simulink model "six_plus_six_AcmsteeringV09_main_1lf"  (R2014a)
settings: Solver=FixedStepDiscrete  StartTime=0.0  StopTime=10.0  FixedStep=0.0005  RelTol=1e-3
InitFcn:
  | Veh_Par_wxt
undefined symbols (not defined in the file or in its folder): acc_spdctl, ag_thr, B, bra_em, bra_pre_gz2, bra_pre_gz34, bra_pre_yd, brakepre_dem_data, brakeTrq_dem_data, bratrq_max, ecucoder_acal, eff_tran, ESP_switch, G, guzhang_lf, guzhang_lm, guzhang_lr, guzhang_rf, guzhang_rm, guzhang_rr, kd1, kd2, ki1, ki2, kp1, kp2, L, myFIS, premax, Radius, RC_switch, s_opt_yi, s_opt_zhuan, s_opt_zhuan_add, s_opt_zhuan_table, spd_map_mot, spd_spdctl, speed_thr_park, TCS_switch, tras_ratio, trq_map_mot, trqmax_yd, trqmax_zx, trqmaxneg, v_gain, v_table, v_thr_park, zhidong_bianmazhi, zhidong_down, zhidong_up, zhidong_youmen, zhuanxiang_bianmazhi, zhuanxiang_down, zhuanxiang_up, zhuanxiang_youmen
libraries: simulink x980, ec5744lib x59, fuzblock x2
(part 5 of 25)

== system six_plus_six_AcmsteeringV09_main_1lf/Data_input/BMS1-2/BMS1 ==
  input : Inport
  Enable : EnablePort
  BMS1_SOC_Ad : Sum
  BMS1_SOC_Convert : DataTypeConversion  OutDataTypeStr=uint32
  BMS1_SOC_F : Gain  Gain=0.1
  BMS1_SOC_L : simulink/Logic and Bit Operations/Bitwise Operator  logicop=AND  UseBitMask=on  BitMask=65535  BitMaskRealWorld=Stored Integer
  BMS1_SOC_O : Constant  Value=0  OutDataTypeStr=single
  BMS1_SOC_S : ArithShift
  BMS1_SOC_Sub : Subsystem
  BMS1_SOC_sat : Saturate  UpperLimit=1000  LowerLimit=0
  BMS1_SOCcv : DataTypeConversion
  BMS1_SOCinput5_Ad : Sum
  BMS1_SOCinput5_C : Constant  Value=256
  BMS1_SOCinput5_P : Product
  BMS1_Sys_Status1_Ad : Sum
  BMS1_Sys_Status1_Convert : DataTypeConversion  OutDataTypeStr=uint32
  BMS1_Sys_Status1_F : Gain
  BMS1_Sys_Status1_L : simulink/Logic and Bit Operations/Bitwise Operator  logicop=AND  UseBitMask=on  BitMask=255  BitMaskRealWorld=Stored Integer
  BMS1_Sys_Status1_O : Constant  Value=0  OutDataTypeStr=single
  BMS1_Sys_Status1_S : ArithShift
  BMS1_Sys_Status1_Sub : Subsystem
  BMS1_Sys_Status1_sat : Saturate  UpperLimit=255  LowerLimit=0
  BMS1_Sys_Status1cv : DataTypeConversion
  BMS1_Sys_Status2_Ad : Sum
  BMS1_Sys_Status2_Convert : DataTypeConversion  OutDataTypeStr=uint32
  BMS1_Sys_Status2_F : Gain
  BMS1_Sys_Status2_L : simulink/Logic and Bit Operations/Bitwise Operator  logicop=AND  UseBitMask=on  BitMask=255  BitMaskRealWorld=Stored Integer
  BMS1_Sys_Status2_O : Constant  Value=0  OutDataTypeStr=single
  BMS1_Sys_Status2_S : ArithShift
  BMS1_Sys_Status2_Sub : Subsystem
  BMS1_Sys_Status2_sat : Saturate  UpperLimit=255  LowerLimit=0
  BMS1_Sys_Status2cv : DataTypeConversion
  BMS1_TotalCurrent_Ad : Sum
  BMS1_TotalCurrent_Convert : DataTypeConversion  OutDataTypeStr=uint32
  BMS1_TotalCurrent_F : Gain  Gain=0.1
  BMS1_TotalCurrent_L : simulink/Logic and Bit Operations/Bitwise Operator  logicop=AND  UseBitMask=on  BitMask=65535  BitMaskRealWorld=Stored Integer
  BMS1_TotalCurrent_O : Constant  Value=-32000  OutDataTypeStr=single
  BMS1_TotalCurrent_S : ArithShift
  BMS1_TotalCurrent_Sub : Subsystem
  BMS1_TotalCurrent_sat : Saturate  UpperLimit=3353.5  LowerLimit=-32000
  BMS1_TotalCurrentcv : DataTypeConversion
  BMS1_TotalCurrentinput3_Ad : Sum
  BMS1_TotalCurrentinput3_C : Constant  Value=256
  BMS1_TotalCurrentinput3_P : Product
  BMS1_TotalVol_Ad : Sum
  BMS1_TotalVol_Convert : DataTypeConversion  OutDataTypeStr=uint32
  BMS1_TotalVol_F : Gain  Gain=0.1
  BMS1_TotalVol_L : simulink/Logic and Bit Operations/Bitwise Operator  logicop=AND  UseBitMask=on  BitMask=65535  BitMaskRealWorld=Stored Integer
  BMS1_TotalVol_O : Constant  Value=0  OutDataTypeStr=single
  BMS1_TotalVol_S : ArithShift
  BMS1_TotalVol_Sub : Subsystem
  BMS1_TotalVol_sat : Saturate  UpperLimit=6553.5  LowerLimit=0
  BMS1_TotalVolcv : DataTypeConversion
  BMS1_TotalVolinput1_Ad : Sum
  BMS1_TotalVolinput1_C : Constant  Value=256
  BMS1_TotalVolinput1_P : Product
  Demux : Demux  Outputs=8
  BMS1_TotalVol_Out : Outport
  BMS1_TotalCurrent_Out : Outport  Port=2
  BMS1_Sys_Status2_Out : Outport  Port=3
  BMS1_Sys_Status1_Out : Outport  Port=4
  BMS1_SOC_Out : Outport  Port=5
  wires:
  BMS1_TotalVol_F/1 -> BMS1_TotalVol_Ad/1
  BMS1_TotalVol_O/1 -> BMS1_TotalVol_Ad/2
  BMS1_TotalVol_Ad/1 -> BMS1_TotalVol_sat/1
  BMS1_TotalVol_sat/1 -> BMS1_TotalVol_Out/1
  Demux/1 -> BMS1_TotalVolinput1_P/1
  BMS1_TotalVolinput1_C/1 -> BMS1_TotalVolinput1_P/2
  BMS1_TotalVolinput1_P/1 -> BMS1_TotalVolinput1_Ad/1
  Demux/2 -> BMS1_TotalVolinput1_Ad/2
  BMS1_TotalVolinput1_Ad/1 -> BMS1_TotalVol_Sub/1(In1)
  BMS1_TotalVol_Sub/1(Out1) -> BMS1_TotalVol_Convert/1
  BMS1_TotalVol_Convert/1 -> BMS1_TotalVol_L/1
  BMS1_TotalVol_L/1 -> BMS1_TotalVol_S/1
  BMS1_TotalVol_S/1 -> BMS1_TotalVolcv/1
  BMS1_TotalVolcv/1 -> BMS1_TotalVol_F/1
  BMS1_TotalCurrent_F/1 -> BMS1_TotalCurrent_Ad/1
  BMS1_TotalCurrent_O/1 -> BMS1_TotalCurrent_Ad/2
  BMS1_TotalCurrent_Ad/1 -> BMS1_TotalCurrent_sat/1
  BMS1_TotalCurrent_sat/1 -> BMS1_TotalCurrent_Out/1
  Demux/3 -> BMS1_TotalCurrentinput3_P/1
  BMS1_TotalCurrentinput3_C/1 -> BMS1_TotalCurrentinput3_P/2
  BMS1_TotalCurrentinput3_P/1 -> BMS1_TotalCurrentinput3_Ad/1
  Demux/4 -> BMS1_TotalCurrentinput3_Ad/2
  BMS1_TotalCurrentinput3_Ad/1 -> BMS1_TotalCurrent_Sub/1(In1)
  BMS1_TotalCurrent_Sub/1(Out1) -> BMS1_TotalCurrent_Convert/1
  BMS1_TotalCurrent_Convert/1 -> BMS1_TotalCurrent_L/1
  BMS1_TotalCurrent_L/1 -> BMS1_TotalCurrent_S/1
  BMS1_TotalCurrent_S/1 -> BMS1_TotalCurrentcv/1
  BMS1_TotalCurrentcv/1 -> BMS1_TotalCurrent_F/1
  BMS1_Sys_Status2_F/1 -> BMS1_Sys_Status2_Ad/1
  BMS1_Sys_Status2_O/1 -> BMS1_Sys_Status2_Ad/2
  BMS1_Sys_Status2_Ad/1 -> BMS1_Sys_Status2_sat/1
  BMS1_Sys_Status2_sat/1 -> BMS1_Sys_Status2_Out/1
  Demux/8 -> BMS1_Sys_Status2_Sub/1(In1)
  BMS1_Sys_Status2_Sub/1(Out1) -> BMS1_Sys_Status2_Convert/1
  BMS1_Sys_Status2_Convert/1 -> BMS1_Sys_Status2_L/1
  BMS1_Sys_Status2_L/1 -> BMS1_Sys_Status2_S/1
  BMS1_Sys_Status2_S/1 -> BMS1_Sys_Status2cv/1
  BMS1_Sys_Status2cv/1 -> BMS1_Sys_Status2_F/1
  BMS1_Sys_Status1_F/1 -> BMS1_Sys_Status1_Ad/1
  BMS1_Sys_Status1_O/1 -> BMS1_Sys_Status1_Ad/2
  BMS1_Sys_Status1_Ad/1 -> BMS1_Sys_Status1_sat/1
  BMS1_Sys_Status1_sat/1 -> BMS1_Sys_Status1_Out/1
  Demux/7 -> BMS1_Sys_Status1_Sub/1(In1)
  BMS1_Sys_Status1_Sub/1(Out1) -> BMS1_Sys_Status1_Convert/1
  BMS1_Sys_Status1_Convert/1 -> BMS1_Sys_Status1_L/1
  BMS1_Sys_Status1_L/1 -> BMS1_Sys_Status1_S/1
  BMS1_Sys_Status1_S/1 -> BMS1_Sys_Status1cv/1
  BMS1_Sys_Status1cv/1 -> BMS1_Sys_Status1_F/1
  BMS1_SOC_F/1 -> BMS1_SOC_Ad/1
  BMS1_SOC_O/1 -> BMS1_SOC_Ad/2
  BMS1_SOC_Ad/1 -> BMS1_SOC_sat/1
  BMS1_SOC_sat/1 -> BMS1_SOC_Out/1
  Demux/5 -> BMS1_SOCinput5_P/1
  BMS1_SOCinput5_C/1 -> BMS1_SOCinput5_P/2
  BMS1_SOCinput5_P/1 -> BMS1_SOCinput5_Ad/1
  Demux/6 -> BMS1_SOCinput5_Ad/2
  BMS1_SOCinput5_Ad/1 -> BMS1_SOC_Sub/1(In1)
  BMS1_SOC_Sub/1(Out1) -> BMS1_SOC_Convert/1
  BMS1_SOC_Convert/1 -> BMS1_SOC_L/1
  BMS1_SOC_L/1 -> BMS1_SOC_S/1
  BMS1_SOC_S/1 -> BMS1_SOCcv/1
  BMS1_SOCcv/1 -> BMS1_SOC_F/1
  input/1 -> Demux/1

== system six_plus_six_AcmsteeringV09_main_1lf/Data_input/BMS1_1/BMS1 ==
  input : Inport
  Enable : EnablePort
  BMS1_SOC_Ad : Sum
  BMS1_SOC_Convert : DataTypeConversion  OutDataTypeStr=uint32
  BMS1_SOC_F : Gain  Gain=0.1
  BMS1_SOC_L : simulink/Logic and Bit Operations/Bitwise Operator  logicop=AND  UseBitMask=on  BitMask=65535  BitMaskRealWorld=Stored Integer
  BMS1_SOC_O : Constant  Value=0  OutDataTypeStr=single
  BMS1_SOC_S : ArithShift
  BMS1_SOC_Sub : Subsystem
  BMS1_SOC_sat : Saturate  UpperLimit=1000  LowerLimit=0
  BMS1_SOCcv : DataTypeConversion
  BMS1_SOCinput5_Ad : Sum
  BMS1_SOCinput5_C : Constant  Value=256
  BMS1_SOCinput5_P : Product
  BMS1_Sys_Status1_Ad : Sum
  BMS1_Sys_Status1_Convert : DataTypeConversion  OutDataTypeStr=uint32
  BMS1_Sys_Status1_F : Gain
  BMS1_Sys_Status1_L : simulink/Logic and Bit Operations/Bitwise Operator  logicop=AND  UseBitMask=on  BitMask=255  BitMaskRealWorld=Stored Integer
  BMS1_Sys_Status1_O : Constant  Value=0  OutDataTypeStr=single
  BMS1_Sys_Status1_S : ArithShift
  BMS1_Sys_Status1_Sub : Subsystem
  BMS1_Sys_Status1_sat : Saturate  UpperLimit=255  LowerLimit=0
  BMS1_Sys_Status1cv : DataTypeConversion
  BMS1_Sys_Status2_Ad : Sum
  BMS1_Sys_Status2_Convert : DataTypeConversion  OutDataTypeStr=uint32
  BMS1_Sys_Status2_F : Gain
  BMS1_Sys_Status2_L : simulink/Logic and Bit Operations/Bitwise Operator  logicop=AND  UseBitMask=on  BitMask=255  BitMaskRealWorld=Stored Integer
  BMS1_Sys_Status2_O : Constant  Value=0  OutDataTypeStr=single
  BMS1_Sys_Status2_S : ArithShift
  BMS1_Sys_Status2_Sub : Subsystem
  BMS1_Sys_Status2_sat : Saturate  UpperLimit=255  LowerLimit=0
  BMS1_Sys_Status2cv : DataTypeConversion
  BMS1_TotalCurrent_Ad : Sum
  BMS1_TotalCurrent_Convert : DataTypeConversion  OutDataTypeStr=uint32
  BMS1_TotalCurrent_F : Gain  Gain=0.1
  BMS1_TotalCurrent_L : simulink/Logic and Bit Operations/Bitwise Operator  logicop=AND  UseBitMask=on  BitMask=65535  BitMaskRealWorld=Stored Integer
  BMS1_TotalCurrent_O : Constant  Value=-32000  OutDataTypeStr=single
  BMS1_TotalCurrent_S : ArithShift
  BMS1_TotalCurrent_Sub : Subsystem
  BMS1_TotalCurrent_sat : Saturate  UpperLimit=3353.5  LowerLimit=-32000
  BMS1_TotalCurrentcv : DataTypeConversion
  BMS1_TotalCurrentinput3_Ad : Sum
  BMS1_TotalCurrentinput3_C : Constant  Value=256
  BMS1_TotalCurrentinput3_P : Product
  BMS1_TotalVol_Ad : Sum
  BMS1_TotalVol_Convert : DataTypeConversion  OutDataTypeStr=uint32
  BMS1_TotalVol_F : Gain  Gain=0.1
  BMS1_TotalVol_L : simulink/Logic and Bit Operations/Bitwise Operator  logicop=AND  UseBitMask=on  BitMask=65535  BitMaskRealWorld=Stored Integer
  BMS1_TotalVol_O : Constant  Value=0  OutDataTypeStr=single
  BMS1_TotalVol_S : ArithShift
  BMS1_TotalVol_Sub : Subsystem
  BMS1_TotalVol_sat : Saturate  UpperLimit=6553.5  LowerLimit=0
  BMS1_TotalVolcv : DataTypeConversion
  BMS1_TotalVolinput1_Ad : Sum
  BMS1_TotalVolinput1_C : Constant  Value=256
  BMS1_TotalVolinput1_P : Product
  Demux : Demux  Outputs=8
  BMS1_TotalVol_Out : Outport
  BMS1_TotalCurrent_Out : Outport  Port=2
  BMS1_Sys_Status2_Out : Outport  Port=3
  BMS1_Sys_Status1_Out : Outport  Port=4
  BMS1_SOC_Out : Outport  Port=5
  wires:
  BMS1_TotalVol_F/1 -> BMS1_TotalVol_Ad/1
  BMS1_TotalVol_O/1 -> BMS1_TotalVol_Ad/2
  BMS1_TotalVol_Ad/1 -> BMS1_TotalVol_sat/1
  BMS1_TotalVol_sat/1 -> BMS1_TotalVol_Out/1
  Demux/1 -> BMS1_TotalVolinput1_P/1
  BMS1_TotalVolinput1_C/1 -> BMS1_TotalVolinput1_P/2
  BMS1_TotalVolinput1_P/1 -> BMS1_TotalVolinput1_Ad/1
  Demux/2 -> BMS1_TotalVolinput1_Ad/2
  BMS1_TotalVolinput1_Ad/1 -> BMS1_TotalVol_Sub/1(In1)
  BMS1_TotalVol_Sub/1(Out1) -> BMS1_TotalVol_Convert/1
  BMS1_TotalVol_Convert/1 -> BMS1_TotalVol_L/1
  BMS1_TotalVol_L/1 -> BMS1_TotalVol_S/1
  BMS1_TotalVol_S/1 -> BMS1_TotalVolcv/1
  BMS1_TotalVolcv/1 -> BMS1_TotalVol_F/1
  BMS1_TotalCurrent_F/1 -> BMS1_TotalCurrent_Ad/1
  BMS1_TotalCurrent_O/1 -> BMS1_TotalCurrent_Ad/2
  BMS1_TotalCurrent_Ad/1 -> BMS1_TotalCurrent_sat/1
  BMS1_TotalCurrent_sat/1 -> BMS1_TotalCurrent_Out/1
  Demux/3 -> BMS1_TotalCurrentinput3_P/1
  BMS1_TotalCurrentinput3_C/1 -> BMS1_TotalCurrentinput3_P/2
  BMS1_TotalCurrentinput3_P/1 -> BMS1_TotalCurrentinput3_Ad/1
  Demux/4 -> BMS1_TotalCurrentinput3_Ad/2
  BMS1_TotalCurrentinput3_Ad/1 -> BMS1_TotalCurrent_Sub/1(In1)
  BMS1_TotalCurrent_Sub/1(Out1) -> BMS1_TotalCurrent_Convert/1
  BMS1_TotalCurrent_Convert/1 -> BMS1_TotalCurrent_L/1
  BMS1_TotalCurrent_L/1 -> BMS1_TotalCurrent_S/1
  BMS1_TotalCurrent_S/1 -> BMS1_TotalCurrentcv/1
  BMS1_TotalCurrentcv/1 -> BMS1_TotalCurrent_F/1
  BMS1_Sys_Status2_F/1 -> BMS1_Sys_Status2_Ad/1
  BMS1_Sys_Status2_O/1 -> BMS1_Sys_Status2_Ad/2
  BMS1_Sys_Status2_Ad/1 -> BMS1_Sys_Status2_sat/1
  BMS1_Sys_Status2_sat/1 -> BMS1_Sys_Status2_Out/1
  Demux/8 -> BMS1_Sys_Status2_Sub/1(In1)
  BMS1_Sys_Status2_Sub/1(Out1) -> BMS1_Sys_Status2_Convert/1
  BMS1_Sys_Status2_Convert/1 -> BMS1_Sys_Status2_L/1
  BMS1_Sys_Status2_L/1 -> BMS1_Sys_Status2_S/1
  BMS1_Sys_Status2_S/1 -> BMS1_Sys_Status2cv/1
  BMS1_Sys_Status2cv/1 -> BMS1_Sys_Status2_F/1
  BMS1_Sys_Status1_F/1 -> BMS1_Sys_Status1_Ad/1
  BMS1_Sys_Status1_O/1 -> BMS1_Sys_Status1_Ad/2
  BMS1_Sys_Status1_Ad/1 -> BMS1_Sys_Status1_sat/1
  BMS1_Sys_Status1_sat/1 -> BMS1_Sys_Status1_Out/1
  Demux/7 -> BMS1_Sys_Status1_Sub/1(In1)
  BMS1_Sys_Status1_Sub/1(Out1) -> BMS1_Sys_Status1_Convert/1
  BMS1_Sys_Status1_Convert/1 -> BMS1_Sys_Status1_L/1
  BMS1_Sys_Status1_L/1 -> BMS1_Sys_Status1_S/1
  BMS1_Sys_Status1_S/1 -> BMS1_Sys_Status1cv/1
  BMS1_Sys_Status1cv/1 -> BMS1_Sys_Status1_F/1
  BMS1_SOC_F/1 -> BMS1_SOC_Ad/1
  BMS1_SOC_O/1 -> BMS1_SOC_Ad/2
  BMS1_SOC_Ad/1 -> BMS1_SOC_sat/1
  BMS1_SOC_sat/1 -> BMS1_SOC_Out/1
  Demux/5 -> BMS1_SOCinput5_P/1
  BMS1_SOCinput5_C/1 -> BMS1_SOCinput5_P/2
  BMS1_SOCinput5_P/1 -> BMS1_SOCinput5_Ad/1
  Demux/6 -> BMS1_SOCinput5_Ad/2
  BMS1_SOCinput5_Ad/1 -> BMS1_SOC_Sub/1(In1)
  BMS1_SOC_Sub/1(Out1) -> BMS1_SOC_Convert/1
  BMS1_SOC_Convert/1 -> BMS1_SOC_L/1
  BMS1_SOC_L/1 -> BMS1_SOC_S/1
  BMS1_SOC_S/1 -> BMS1_SOCcv/1
  BMS1_SOCcv/1 -> BMS1_SOC_F/1
  input/1 -> Demux/1

== system six_plus_six_AcmsteeringV09_main_1lf/Data_input/BMS2/BMS2 ==
  input : Inport
  Enable : EnablePort
  BMS2_HighSingleVol_Ad : Sum
  BMS2_HighSingleVol_Convert : DataTypeConversion  OutDataTypeStr=uint32
  BMS2_HighSingleVol_F : Gain
  BMS2_HighSingleVol_L : simulink/Logic and Bit Operations/Bitwise Operator  logicop=AND  UseBitMask=on  BitMask=65535  BitMaskRealWorld=Stored Integer
  BMS2_HighSingleVol_O : Constant  Value=0  OutDataTypeStr=single
  BMS2_HighSingleVol_S : ArithShift
  BMS2_HighSingleVol_Sub : Subsystem
  BMS2_HighSingleVol_sat : Saturate  UpperLimit=10  LowerLimit=0
  BMS2_HighSingleVolcv : DataTypeConversion
  BMS2_HighSingleVolinput1_Ad : Sum
  BMS2_HighSingleVolinput1_C : Constant  Value=256
  BMS2_HighSingleVolinput1_P : Product
  BMS2_LowSingleVol_Ad : Sum
  BMS2_LowSingleVol_Convert : DataTypeConversion  OutDataTypeStr=uint32
  BMS2_LowSingleVol_F : Gain
  BMS2_LowSingleVol_L : simulink/Logic and Bit Operations/Bitwise Operator  logicop=AND  UseBitMask=on  BitMask=65535  BitMaskRealWorld=Stored Integer
  BMS2_LowSingleVol_O : Constant  Value=0  OutDataTypeStr=single
  BMS2_LowSingleVol_S : ArithShift
  BMS2_LowSingleVol_Sub : Subsystem
  BMS2_LowSingleVol_sat : Saturate  UpperLimit=65535  LowerLimit=0
  BMS2_LowSingleVolcv : DataTypeConversion
  BMS2_LowSingleVolinput3_Ad : Sum
  BMS2_LowSingleVolinput3_C : Constant  Value=256
  BMS2_LowSingleVolinput3_P : Product
  Demux : Demux  Outputs=8
  BMS2_LowSingleVol_Out : Outport
  BMS2_HighSingleVol_Out : Outport  Port=2
  wires:
  BMS2_LowSingleVol_F/1 -> BMS2_LowSingleVol_Ad/1
  BMS2_LowSingleVol_O/1 -> BMS2_LowSingleVol_Ad/2
  BMS2_LowSingleVol_Ad/1 -> BMS2_LowSingleVol_sat/1
  BMS2_LowSingleVol_sat/1 -> BMS2_LowSingleVol_Out/1
  Demux/3 -> BMS2_LowSingleVolinput3_P/1
  BMS2_LowSingleVolinput3_C/1 -> BMS2_LowSingleVolinput3_P/2
  BMS2_LowSingleVolinput3_P/1 -> BMS2_LowSingleVolinput3_Ad/1
  Demux/4 -> BMS2_LowSingleVolinput3_Ad/2
  BMS2_LowSingleVolinput3_Ad/1 -> BMS2_LowSingleVol_Sub/1(In1)
  BMS2_LowSingleVol_Sub/1(Out1) -> BMS2_LowSingleVol_Convert/1
  BMS2_LowSingleVol_Convert/1 -> BMS2_LowSingleVol_L/1
  BMS2_LowSingleVol_L/1 -> BMS2_LowSingleVol_S/1
  BMS2_LowSingleVol_S/1 -> BMS2_LowSingleVolcv/1
  BMS2_LowSingleVolcv/1 -> BMS2_LowSingleVol_F/1
  BMS2_HighSingleVol_F/1 -> BMS2_HighSingleVol_Ad/1
  BMS2_HighSingleVol_O/1 -> BMS2_HighSingleVol_Ad/2
  BMS2_HighSingleVol_Ad/1 -> BMS2_HighSingleVol_sat/1
  BMS2_HighSingleVol_sat/1 -> BMS2_HighSingleVol_Out/1
  Demux/1 -> BMS2_HighSingleVolinput1_P/1
  BMS2_HighSingleVolinput1_C/1 -> BMS2_HighSingleVolinput1_P/2
  BMS2_HighSingleVolinput1_P/1 -> BMS2_HighSingleVolinput1_Ad/1
  Demux/2 -> BMS2_HighSingleVolinput1_Ad/2
  BMS2_HighSingleVolinput1_Ad/1 -> BMS2_HighSingleVol_Sub/1(In1)
  BMS2_HighSingleVol_Sub/1(Out1) -> BMS2_HighSingleVol_Convert/1
  BMS2_HighSingleVol_Convert/1 -> BMS2_HighSingleVol_L/1
  BMS2_HighSingleVol_L/1 -> BMS2_HighSingleVol_S/1
  BMS2_HighSingleVol_S/1 -> BMS2_HighSingleVolcv/1
  BMS2_HighSingleVolcv/1 -> BMS2_HighSingleVol_F/1
  input/1 -> Demux/1

== system six_plus_six_AcmsteeringV09_main_1lf/Data_input/BMS2_1/BMS2 ==
  input : Inport
  Enable : EnablePort
  BMS2_HighSingleVol_Ad : Sum
  BMS2_HighSingleVol_Convert : DataTypeConversion  OutDataTypeStr=uint32
  BMS2_HighSingleVol_F : Gain
  BMS2_HighSingleVol_L : simulink/Logic and Bit Operations/Bitwise Operator  logicop=AND  UseBitMask=on  BitMask=65535  BitMaskRealWorld=Stored Integer
  BMS2_HighSingleVol_O : Constant  Value=0  OutDataTypeStr=single
  BMS2_HighSingleVol_S : ArithShift
  BMS2_HighSingleVol_Sub : Subsystem
  BMS2_HighSingleVol_sat : Saturate  UpperLimit=10  LowerLimit=0
  BMS2_HighSingleVolcv : DataTypeConversion
  BMS2_HighSingleVolinput1_Ad : Sum
  BMS2_HighSingleVolinput1_C : Constant  Value=256
  BMS2_HighSingleVolinput1_P : Product
  BMS2_LowSingleVol_Ad : Sum
  BMS2_LowSingleVol_Convert : DataTypeConversion  OutDataTypeStr=uint32
  BMS2_LowSingleVol_F : Gain
  BMS2_LowSingleVol_L : simulink/Logic and Bit Operations/Bitwise Operator  logicop=AND  UseBitMask=on  BitMask=65535  BitMaskRealWorld=Stored Integer
  BMS2_LowSingleVol_O : Constant  Value=0  OutDataTypeStr=single
  BMS2_LowSingleVol_S : ArithShift
  BMS2_LowSingleVol_Sub : Subsystem
  BMS2_LowSingleVol_sat : Saturate  UpperLimit=65535  LowerLimit=0
  BMS2_LowSingleVolcv : DataTypeConversion
  BMS2_LowSingleVolinput3_Ad : Sum
  BMS2_LowSingleVolinput3_C : Constant  Value=256
  BMS2_LowSingleVolinput3_P : Product
  Demux : Demux  Outputs=8
  BMS2_LowSingleVol_Out : Outport
  BMS2_HighSingleVol_Out : Outport  Port=2
  wires:
  BMS2_LowSingleVol_F/1 -> BMS2_LowSingleVol_Ad/1
  BMS2_LowSingleVol_O/1 -> BMS2_LowSingleVol_Ad/2
  BMS2_LowSingleVol_Ad/1 -> BMS2_LowSingleVol_sat/1
  BMS2_LowSingleVol_sat/1 -> BMS2_LowSingleVol_Out/1
  Demux/3 -> BMS2_LowSingleVolinput3_P/1
  BMS2_LowSingleVolinput3_C/1 -> BMS2_LowSingleVolinput3_P/2
  BMS2_LowSingleVolinput3_P/1 -> BMS2_LowSingleVolinput3_Ad/1
  Demux/4 -> BMS2_LowSingleVolinput3_Ad/2
  BMS2_LowSingleVolinput3_Ad/1 -> BMS2_LowSingleVol_Sub/1(In1)
  BMS2_LowSingleVol_Sub/1(Out1) -> BMS2_LowSingleVol_Convert/1
  BMS2_LowSingleVol_Convert/1 -> BMS2_LowSingleVol_L/1
  BMS2_LowSingleVol_L/1 -> BMS2_LowSingleVol_S/1
  BMS2_LowSingleVol_S/1 -> BMS2_LowSingleVolcv/1
  BMS2_LowSingleVolcv/1 -> BMS2_LowSingleVol_F/1
  BMS2_HighSingleVol_F/1 -> BMS2_HighSingleVol_Ad/1
  BMS2_HighSingleVol_O/1 -> BMS2_HighSingleVol_Ad/2
  BMS2_HighSingleVol_Ad/1 -> BMS2_HighSingleVol_sat/1
  BMS2_HighSingleVol_sat/1 -> BMS2_HighSingleVol_Out/1
  Demux/1 -> BMS2_HighSingleVolinput1_P/1
  BMS2_HighSingleVolinput1_C/1 -> BMS2_HighSingleVolinput1_P/2
  BMS2_HighSingleVolinput1_P/1 -> BMS2_HighSingleVolinput1_Ad/1
  Demux/2 -> BMS2_HighSingleVolinput1_Ad/2
  BMS2_HighSingleVolinput1_Ad/1 -> BMS2_HighSingleVol_Sub/1(In1)
  BMS2_HighSingleVol_Sub/1(Out1) -> BMS2_HighSingleVol_Convert/1
  BMS2_HighSingleVol_Convert/1 -> BMS2_HighSingleVol_L/1
  BMS2_HighSingleVol_L/1 -> BMS2_HighSingleVol_S/1
  BMS2_HighSingleVol_S/1 -> BMS2_HighSingleVolcv/1
  BMS2_HighSingleVolcv/1 -> BMS2_HighSingleVol_F/1
  input/1 -> Demux/1

== system six_plus_six_AcmsteeringV09_main_1lf/Data_input/BMS2_2/BMS2 ==
  input : Inport
  Enable : EnablePort
  BMS2_HighSingleVol_Ad : Sum
  BMS2_HighSingleVol_Convert : DataTypeConversion  OutDataTypeStr=uint32
  BMS2_HighSingleVol_F : Gain
  BMS2_HighSingleVol_L : simulink/Logic and Bit Operations/Bitwise Operator  logicop=AND  UseBitMask=on  BitMask=65535  BitMaskRealWorld=Stored Integer
  BMS2_HighSingleVol_O : Constant  Value=0  OutDataTypeStr=single
  BMS2_HighSingleVol_S : ArithShift
  BMS2_HighSingleVol_Sub : Subsystem
  BMS2_HighSingleVol_sat : Saturate  UpperLimit=10  LowerLimit=0
  BMS2_HighSingleVolcv : DataTypeConversion
  BMS2_HighSingleVolinput1_Ad : Sum
  BMS2_HighSingleVolinput1_C : Constant  Value=256
  BMS2_HighSingleVolinput1_P : Product
  BMS2_LowSingleVol_Ad : Sum
  BMS2_LowSingleVol_Convert : DataTypeConversion  OutDataTypeStr=uint32
  BMS2_LowSingleVol_F : Gain
  BMS2_LowSingleVol_L : simulink/Logic and Bit Operations/Bitwise Operator  logicop=AND  UseBitMask=on  BitMask=65535  BitMaskRealWorld=Stored Integer
  BMS2_LowSingleVol_O : Constant  Value=0  OutDataTypeStr=single
  BMS2_LowSingleVol_S : ArithShift
  BMS2_LowSingleVol_Sub : Subsystem
  BMS2_LowSingleVol_sat : Saturate  UpperLimit=65535  LowerLimit=0
  BMS2_LowSingleVolcv : DataTypeConversion
  BMS2_LowSingleVolinput3_Ad : Sum
  BMS2_LowSingleVolinput3_C : Constant  Value=256
  BMS2_LowSingleVolinput3_P : Product
  Demux : Demux  Outputs=8
  BMS2_LowSingleVol_Out : Outport
  BMS2_HighSingleVol_Out : Outport  Port=2
  wires:
  BMS2_LowSingleVol_F/1 -> BMS2_LowSingleVol_Ad/1
  BMS2_LowSingleVol_O/1 -> BMS2_LowSingleVol_Ad/2
  BMS2_LowSingleVol_Ad/1 -> BMS2_LowSingleVol_sat/1
  BMS2_LowSingleVol_sat/1 -> BMS2_LowSingleVol_Out/1
  Demux/3 -> BMS2_LowSingleVolinput3_P/1
  BMS2_LowSingleVolinput3_C/1 -> BMS2_LowSingleVolinput3_P/2
  BMS2_LowSingleVolinput3_P/1 -> BMS2_LowSingleVolinput3_Ad/1
  Demux/4 -> BMS2_LowSingleVolinput3_Ad/2
  BMS2_LowSingleVolinput3_Ad/1 -> BMS2_LowSingleVol_Sub/1(In1)
  BMS2_LowSingleVol_Sub/1(Out1) -> BMS2_LowSingleVol_Convert/1
  BMS2_LowSingleVol_Convert/1 -> BMS2_LowSingleVol_L/1
  BMS2_LowSingleVol_L/1 -> BMS2_LowSingleVol_S/1
  BMS2_LowSingleVol_S/1 -> BMS2_LowSingleVolcv/1
  BMS2_LowSingleVolcv/1 -> BMS2_LowSingleVol_F/1
  BMS2_HighSingleVol_F/1 -> BMS2_HighSingleVol_Ad/1
  BMS2_HighSingleVol_O/1 -> BMS2_HighSingleVol_Ad/2
  BMS2_HighSingleVol_Ad/1 -> BMS2_HighSingleVol_sat/1
  BMS2_HighSingleVol_sat/1 -> BMS2_HighSingleVol_Out/1
  Demux/1 -> BMS2_HighSingleVolinput1_P/1
  BMS2_HighSingleVolinput1_C/1 -> BMS2_HighSingleVolinput1_P/2
  BMS2_HighSingleVolinput1_P/1 -> BMS2_HighSingleVolinput1_Ad/1
  Demux/2 -> BMS2_HighSingleVolinput1_Ad/2
  BMS2_HighSingleVolinput1_Ad/1 -> BMS2_HighSingleVol_Sub/1(In1)
  BMS2_HighSingleVol_Sub/1(Out1) -> BMS2_HighSingleVol_Convert/1
  BMS2_HighSingleVol_Convert/1 -> BMS2_HighSingleVol_L/1
  BMS2_HighSingleVol_L/1 -> BMS2_HighSingleVol_S/1
  BMS2_HighSingleVol_S/1 -> BMS2_HighSingleVolcv/1
  BMS2_HighSingleVolcv/1 -> BMS2_HighSingleVol_F/1
  input/1 -> Demux/1

== system six_plus_six_AcmsteeringV09_main_1lf/Data_input/BMS3/BMS3 ==
  input : Inport
  Enable : EnablePort
  BMS3_HighTemperature_Ad : Sum
  BMS3_HighTemperature_Convert : DataTypeConversion  OutDataTypeStr=uint32
  BMS3_HighTemperature_F : Gain
  BMS3_HighTemperature_L : simulink/Logic and Bit Operations/Bitwise Operator  logicop=AND  UseBitMask=on  BitMask=255  BitMaskRealWorld=Stored Integer
  BMS3_HighTemperature_O : Constant  Value=-40  OutDataTypeStr=single
  BMS3_HighTemperature_S : ArithShift
  BMS3_HighTemperature_Sub : Subsystem
  BMS3_HighTemperature_sat : Saturate  UpperLimit=210  LowerLimit=-40
  BMS3_HighTemperaturecv : DataTypeConversion
  BMS3_LowTemperature_Ad : Sum
  BMS3_LowTemperature_Convert : DataTypeConversion  OutDataTypeStr=uint32
  BMS3_LowTemperature_F : Gain
  BMS3_LowTemperature_L : simulink/Logic and Bit Operations/Bitwise Operator  logicop=AND  UseBitMask=on  BitMask=255  BitMaskRealWorld=Stored Integer
  BMS3_LowTemperature_O : Constant  Value=-40  OutDataTypeStr=single
  BMS3_LowTemperature_S : ArithShift
  BMS3_LowTemperature_Sub : Subsystem
  BMS3_LowTemperature_sat : Saturate  UpperLimit=210  LowerLimit=-40
  BMS3_LowTemperaturecv : DataTypeConversion
  Demux : Demux  Outputs=8
  BMS3_LowTemperature_Out : Outport
  BMS3_HighTemperature_Out : Outport  Port=2
  wires:
  BMS3_LowTemperature_F/1 -> BMS3_LowTemperature_Ad/1
  BMS3_LowTemperature_O/1 -> BMS3_LowTemperature_Ad/2
  BMS3_LowTemperature_Ad/1 -> BMS3_LowTemperature_sat/1
  BMS3_LowTemperature_sat/1 -> BMS3_LowTemperature_Out/1
  Demux/3 -> BMS3_LowTemperature_Sub/1(In1)
  BMS3_LowTemperature_Sub/1(Out1) -> BMS3_LowTemperature_Convert/1
  BMS3_LowTemperature_Convert/1 -> BMS3_LowTemperature_L/1
  BMS3_LowTemperature_L/1 -> BMS3_LowTemperature_S/1
  BMS3_LowTemperature_S/1 -> BMS3_LowTemperaturecv/1
  BMS3_LowTemperaturecv/1 -> BMS3_LowTemperature_F/1
  BMS3_HighTemperature_F/1 -> BMS3_HighTemperature_Ad/1
  BMS3_HighTemperature_O/1 -> BMS3_HighTemperature_Ad/2
  BMS3_HighTemperature_Ad/1 -> BMS3_HighTemperature_sat/1
  BMS3_HighTemperature_sat/1 -> BMS3_HighTemperature_Out/1
  Demux/1 -> BMS3_HighTemperature_Sub/1(In1)
  BMS3_HighTemperature_Sub/1(Out1) -> BMS3_HighTemperature_Convert/1
  BMS3_HighTemperature_Convert/1 -> BMS3_HighTemperature_L/1
  BMS3_HighTemperature_L/1 -> BMS3_HighTemperature_S/1
  BMS3_HighTemperature_S/1 -> BMS3_HighTemperaturecv/1
  BMS3_HighTemperaturecv/1 -> BMS3_HighTemperature_F/1
  input/1 -> Demux/1

== system six_plus_six_AcmsteeringV09_main_1lf/Data_input/BMS3_1/BMS3 ==
  input : Inport
  Enable : EnablePort
  BMS3_HighTemperature_Ad : Sum
  BMS3_HighTemperature_Convert : DataTypeConversion  OutDataTypeStr=uint32
  BMS3_HighTemperature_F : Gain
  BMS3_HighTemperature_L : simulink/Logic and Bit Operations/Bitwise Operator  logicop=AND  UseBitMask=on  BitMask=255  BitMaskRealWorld=Stored Integer
  BMS3_HighTemperature_O : Constant  Value=-40  OutDataTypeStr=single
  BMS3_HighTemperature_S : ArithShift
  BMS3_HighTemperature_Sub : Subsystem
  BMS3_HighTemperature_sat : Saturate  UpperLimit=210  LowerLimit=-40
  BMS3_HighTemperaturecv : DataTypeConversion
  BMS3_LowTemperature_Ad : Sum
  BMS3_LowTemperature_Convert : DataTypeConversion  OutDataTypeStr=uint32
  BMS3_LowTemperature_F : Gain
  BMS3_LowTemperature_L : simulink/Logic and Bit Operations/Bitwise Operator  logicop=AND  UseBitMask=on  BitMask=255  BitMaskRealWorld=Stored Integer
  BMS3_LowTemperature_O : Constant  Value=-40  OutDataTypeStr=single
  BMS3_LowTemperature_S : ArithShift
  BMS3_LowTemperature_Sub : Subsystem
  BMS3_LowTemperature_sat : Saturate  UpperLimit=210  LowerLimit=-40
  BMS3_LowTemperaturecv : DataTypeConversion
  Demux : Demux  Outputs=8
  BMS3_LowTemperature_Out : Outport
  BMS3_HighTemperature_Out : Outport  Port=2
  wires:
  BMS3_LowTemperature_F/1 -> BMS3_LowTemperature_Ad/1
  BMS3_LowTemperature_O/1 -> BMS3_LowTemperature_Ad/2
  BMS3_LowTemperature_Ad/1 -> BMS3_LowTemperature_sat/1
  BMS3_LowTemperature_sat/1 -> BMS3_LowTemperature_Out/1
  Demux/3 -> BMS3_LowTemperature_Sub/1(In1)
  BMS3_LowTemperature_Sub/1(Out1) -> BMS3_LowTemperature_Convert/1
  BMS3_LowTemperature_Convert/1 -> BMS3_LowTemperature_L/1
  BMS3_LowTemperature_L/1 -> BMS3_LowTemperature_S/1
  BMS3_LowTemperature_S/1 -> BMS3_LowTemperaturecv/1
  BMS3_LowTemperaturecv/1 -> BMS3_LowTemperature_F/1
  BMS3_HighTemperature_F/1 -> BMS3_HighTemperature_Ad/1
  BMS3_HighTemperature_O/1 -> BMS3_HighTemperature_Ad/2
  BMS3_HighTemperature_Ad/1 -> BMS3_HighTemperature_sat/1
  BMS3_HighTemperature_sat/1 -> BMS3_HighTemperature_Out/1
  Demux/1 -> BMS3_HighTemperature_Sub/1(In1)
  BMS3_HighTemperature_Sub/1(Out1) -> BMS3_HighTemperature_Convert/1
  BMS3_HighTemperature_Convert/1 -> BMS3_HighTemperature_L/1
  BMS3_HighTemperature_L/1 -> BMS3_HighTemperature_S/1
  BMS3_HighTemperature_S/1 -> BMS3_HighTemperaturecv/1
  BMS3_HighTemperaturecv/1 -> BMS3_HighTemperature_F/1
  input/1 -> Demux/1

== system six_plus_six_AcmsteeringV09_main_1lf/Data_input/BMS3_2/BMS3 ==
  input : Inport
  Enable : EnablePort
  BMS3_HighTemperature_Ad : Sum
  BMS3_HighTemperature_Convert : DataTypeConversion  OutDataTypeStr=uint32
  BMS3_HighTemperature_F : Gain
  BMS3_HighTemperature_L : simulink/Logic and Bit Operations/Bitwise Operator  logicop=AND  UseBitMask=on  BitMask=255  BitMaskRealWorld=Stored Integer
  BMS3_HighTemperature_O : Constant  Value=-40  OutDataTypeStr=single
  BMS3_HighTemperature_S : ArithShift
  BMS3_HighTemperature_Sub : Subsystem
  BMS3_HighTemperature_sat : Saturate  UpperLimit=210  LowerLimit=-40
  BMS3_HighTemperaturecv : DataTypeConversion
  BMS3_LowTemperature_Ad : Sum
  BMS3_LowTemperature_Convert : DataTypeConversion  OutDataTypeStr=uint32
  BMS3_LowTemperature_F : Gain
  BMS3_LowTemperature_L : simulink/Logic and Bit Operations/Bitwise Operator  logicop=AND  UseBitMask=on  BitMask=255  BitMaskRealWorld=Stored Integer
  BMS3_LowTemperature_O : Constant  Value=-40  OutDataTypeStr=single
  BMS3_LowTemperature_S : ArithShift
  BMS3_LowTemperature_Sub : Subsystem
  BMS3_LowTemperature_sat : Saturate  UpperLimit=210  LowerLimit=-40
  BMS3_LowTemperaturecv : DataTypeConversion
  Demux : Demux  Outputs=8
  BMS3_LowTemperature_Out : Outport
  BMS3_HighTemperature_Out : Outport  Port=2
  wires:
  BMS3_LowTemperature_F/1 -> BMS3_LowTemperature_Ad/1
  BMS3_LowTemperature_O/1 -> BMS3_LowTemperature_Ad/2
  BMS3_LowTemperature_Ad/1 -> BMS3_LowTemperature_sat/1
  BMS3_LowTemperature_sat/1 -> BMS3_LowTemperature_Out/1
  Demux/3 -> BMS3_LowTemperature_Sub/1(In1)
  BMS3_LowTemperature_Sub/1(Out1) -> BMS3_LowTemperature_Convert/1
  BMS3_LowTemperature_Convert/1 -> BMS3_LowTemperature_L/1
  BMS3_LowTemperature_L/1 -> BMS3_LowTemperature_S/1
  BMS3_LowTemperature_S/1 -> BMS3_LowTemperaturecv/1
  BMS3_LowTemperaturecv/1 -> BMS3_LowTemperature_F/1
  BMS3_HighTemperature_F/1 -> BMS3_HighTemperature_Ad/1
  BMS3_HighTemperature_O/1 -> BMS3_HighTemperature_Ad/2
  BMS3_HighTemperature_Ad/1 -> BMS3_HighTemperature_sat/1
  BMS3_HighTemperature_sat/1 -> BMS3_HighTemperature_Out/1
  Demux/1 -> BMS3_HighTemperature_Sub/1(In1)
  BMS3_HighTemperature_Sub/1(Out1) -> BMS3_HighTemperature_Convert/1
  BMS3_HighTemperature_Convert/1 -> BMS3_HighTemperature_L/1
  BMS3_HighTemperature_L/1 -> BMS3_HighTemperature_S/1
  BMS3_HighTemperature_S/1 -> BMS3_HighTemperaturecv/1
  BMS3_HighTemperaturecv/1 -> BMS3_HighTemperature_F/1
  input/1 -> Demux/1

== system six_plus_six_AcmsteeringV09_main_1lf/Data_input/BMS4/BMS4 ==
  input : Inport
  Enable : EnablePort
  BMS4_InputVolACC_Ad : Sum
  BMS4_InputVolACC_Convert : DataTypeConversion  OutDataTypeStr=uint32
  BMS4_InputVolACC_F : Gain  Gain=0.1
  BMS4_InputVolACC_L : simulink/Logic and Bit Operations/Bitwise Operator  logicop=AND  UseBitMask=on  BitMask=65535  BitMaskRealWorld=Stored Integer
  BMS4_InputVolACC_O : Constant  Value=0  OutDataTypeStr=single
  BMS4_InputVolACC_S : ArithShift
  BMS4_InputVolACC_Sub : Subsystem
  BMS4_InputVolACC_sat : Saturate  UpperLimit=6553.5  LowerLimit=0
  BMS4_InputVolACCcv : DataTypeConversion
  BMS4_InputVolACCinput2_Ad : Sum
  BMS4_InputVolACCinput2_C : Constant  Value=256
  BMS4_InputVolACCinput2_P : Product
  BMS4_InputVolCHG_Ad : Sum
  BMS4_InputVolCHG_Convert : DataTypeConversion  OutDataTypeStr=uint32
  BMS4_InputVolCHG_F : Gain  Gain=0.1
  BMS4_InputVolCHG_L : simulink/Logic and Bit Operations/Bitwise Operator  logicop=AND  UseBitMask=on  BitMask=65535  BitMaskRealWorld=Stored Integer
  BMS4_InputVolCHG_O : Constant  Value=0  OutDataTypeStr=single
  BMS4_InputVolCHG_S : ArithShift
  BMS4_InputVolCHG_Sub : Subsystem
  BMS4_InputVolCHG_sat : Saturate  UpperLimit=6553.5  LowerLimit=0
  BMS4_InputVolCHGcv : DataTypeConversion
  BMS4_InputVolCHGinput6_Ad : Sum
  BMS4_InputVolCHGinput6_C : Constant  Value=256
  BMS4_InputVolCHGinput6_P : Product
  BMS4_InputVolKEYON_Ad : Sum
  BMS4_InputVolKEYON_Convert : DataTypeConversion  OutDataTypeStr=uint32
  BMS4_InputVolKEYON_F : Gain  Gain=0.1
  BMS4_InputVolKEYON_L : simulink/Logic and Bit Operations/Bitwise Operator  logicop=AND  UseBitMask=on  BitMask=65535  BitMaskRealWorld=Stored Integer
  BMS4_InputVolKEYON_O : Constant  Value=0  OutDataTypeStr=single
  BMS4_InputVolKEYON_S : ArithShift
  BMS4_InputVolKEYON_Sub : Subsystem
  BMS4_InputVolKEYON_sat : Saturate  UpperLimit=6553.5  LowerLimit=0
  BMS4_InputVolKEYONcv : DataTypeConversion
  BMS4_InputVolKEYONinput4_Ad : Sum
  BMS4_InputVolKEYONinput4_C : Constant  Value=256
  BMS4_InputVolKEYONinput4_P : Product
  BMS4_Sys_Status3_Ad : Sum
  BMS4_Sys_Status3_Convert : DataTypeConversion  OutDataTypeStr=uint32
  BMS4_Sys_Status3_F : Gain
  BMS4_Sys_Status3_L : simulink/Logic and Bit Operations/Bitwise Operator  logicop=AND  UseBitMask=on  BitMask=255  BitMaskRealWorld=Stored Integer
  BMS4_Sys_Status3_O : Constant  Value=0  OutDataTypeStr=single
  BMS4_Sys_Status3_S : ArithShift
  BMS4_Sys_Status3_Sub : Subsystem
  BMS4_Sys_Status3_sat : Saturate  UpperLimit=255  LowerLimit=0
  BMS4_Sys_Status3cv : DataTypeConversion
  Demux : Demux  Outputs=8
  BMS4_Sys_Status3_Out : Outport
  BMS4_InputVolKEYON_Out : Outport  Port=2
  BMS4_InputVolCHG_Out : Outport  Port=3
  BMS4_InputVolACC_Out : Outport  Port=4
  wires:
  BMS4_Sys_Status3_F/1 -> BMS4_Sys_Status3_Ad/1
  BMS4_Sys_Status3_O/1 -> BMS4_Sys_Status3_Ad/2
  BMS4_Sys_Status3_Ad/1 -> BMS4_Sys_Status3_sat/1
  BMS4_Sys_Status3_sat/1 -> BMS4_Sys_Status3_Out/1
  Demux/1 -> BMS4_Sys_Status3_Sub/1(In1)
  BMS4_Sys_Status3_Sub/1(Out1) -> BMS4_Sys_Status3_Convert/1
  BMS4_Sys_Status3_Convert/1 -> BMS4_Sys_Status3_L/1
  BMS4_Sys_Status3_L/1 -> BMS4_Sys_Status3_S/1
  BMS4_Sys_Status3_S/1 -> BMS4_Sys_Status3cv/1
  BMS4_Sys_Status3cv/1 -> BMS4_Sys_Status3_F/1
  BMS4_InputVolKEYON_F/1 -> BMS4_InputVolKEYON_Ad/1
  BMS4_InputVolKEYON_O/1 -> BMS4_InputVolKEYON_Ad/2
  BMS4_InputVolKEYON_Ad/1 -> BMS4_InputVolKEYON_sat/1
  BMS4_InputVolKEYON_sat/1 -> BMS4_InputVolKEYON_Out/1
  Demux/4 -> BMS4_InputVolKEYONinput4_P/1
  BMS4_InputVolKEYONinput4_C/1 -> BMS4_InputVolKEYONinput4_P/2
  BMS4_InputVolKEYONinput4_P/1 -> BMS4_InputVolKEYONinput4_Ad/1
  Demux/5 -> BMS4_InputVolKEYONinput4_Ad/2
  BMS4_InputVolKEYONinput4_Ad/1 -> BMS4_InputVolKEYON_Sub/1(In1)
  BMS4_InputVolKEYON_Sub/1(Out1) -> BMS4_InputVolKEYON_Convert/1
  BMS4_InputVolKEYON_Convert/1 -> BMS4_InputVolKEYON_L/1
  BMS4_InputVolKEYON_L/1 -> BMS4_InputVolKEYON_S/1
  BMS4_InputVolKEYON_S/1 -> BMS4_InputVolKEYONcv/1
  BMS4_InputVolKEYONcv/1 -> BMS4_InputVolKEYON_F/1
  BMS4_InputVolCHG_F/1 -> BMS4_InputVolCHG_Ad/1
  BMS4_InputVolCHG_O/1 -> BMS4_InputVolCHG_Ad/2
  BMS4_InputVolCHG_Ad/1 -> BMS4_InputVolCHG_sat/1
  BMS4_InputVolCHG_sat/1 -> BMS4_InputVolCHG_Out/1
  Demux/6 -> BMS4_InputVolCHGinput6_P/1
  BMS4_InputVolCHGinput6_C/1 -> BMS4_InputVolCHGinput6_P/2
  BMS4_InputVolCHGinput6_P/1 -> BMS4_InputVolCHGinput6_Ad/1
  Demux/7 -> BMS4_InputVolCHGinput6_Ad/2
  BMS4_InputVolCHGinput6_Ad/1 -> BMS4_InputVolCHG_Sub/1(In1)
  BMS4_InputVolCHG_Sub/1(Out1) -> BMS4_InputVolCHG_Convert/1
  BMS4_InputVolCHG_Convert/1 -> BMS4_InputVolCHG_L/1
  BMS4_InputVolCHG_L/1 -> BMS4_InputVolCHG_S/1
  BMS4_InputVolCHG_S/1 -> BMS4_InputVolCHGcv/1
  BMS4_InputVolCHGcv/1 -> BMS4_InputVolCHG_F/1
  BMS4_InputVolACC_F/1 -> BMS4_InputVolACC_Ad/1
  BMS4_InputVolACC_O/1 -> BMS4_InputVolACC_Ad/2
  BMS4_InputVolACC_Ad/1 -> BMS4_InputVolACC_sat/1
  BMS4_InputVolACC_sat/1 -> BMS4_InputVolACC_Out/1
  Demux/2 -> BMS4_InputVolACCinput2_P/1
  BMS4_InputVolACCinput2_C/1 -> BMS4_InputVolACCinput2_P/2
  BMS4_InputVolACCinput2_P/1 -> BMS4_InputVolACCinput2_Ad/1
  Demux/3 -> BMS4_InputVolACCinput2_Ad/2
  BMS4_InputVolACCinput2_Ad/1 -> BMS4_InputVolACC_Sub/1(In1)
  BMS4_InputVolACC_Sub/1(Out1) -> BMS4_InputVolACC_Convert/1
  BMS4_InputVolACC_Convert/1 -> BMS4_InputVolACC_L/1
  BMS4_InputVolACC_L/1 -> BMS4_InputVolACC_S/1
  BMS4_InputVolACC_S/1 -> BMS4_InputVolACCcv/1
  BMS4_InputVolACCcv/1 -> BMS4_InputVolACC_F/1
  input/1 -> Demux/1

== system six_plus_six_AcmsteeringV09_main_1lf/Data_input/BMS4_1/BMS4 ==
  input : Inport
  Enable : EnablePort
  BMS4_InputVolACC_Ad : Sum
  BMS4_InputVolACC_Convert : DataTypeConversion  OutDataTypeStr=uint32
  BMS4_InputVolACC_F : Gain  Gain=0.1
  BMS4_InputVolACC_L : simulink/Logic and Bit Operations/Bitwise Operator  logicop=AND  UseBitMask=on  BitMask=65535  BitMaskRealWorld=Stored Integer
  BMS4_InputVolACC_O : Constant  Value=0  OutDataTypeStr=single
  BMS4_InputVolACC_S : ArithShift
  BMS4_InputVolACC_Sub : Subsystem
  BMS4_InputVolACC_sat : Saturate  UpperLimit=6553.5  LowerLimit=0
  BMS4_InputVolACCcv : DataTypeConversion
  BMS4_InputVolACCinput2_Ad : Sum
  BMS4_InputVolACCinput2_C : Constant  Value=256
  BMS4_InputVolACCinput2_P : Product
  BMS4_InputVolCHG_Ad : Sum
  BMS4_InputVolCHG_Convert : DataTypeConversion  OutDataTypeStr=uint32
  BMS4_InputVolCHG_F : Gain  Gain=0.1
  BMS4_InputVolCHG_L : simulink/Logic and Bit Operations/Bitwise Operator  logicop=AND  UseBitMask=on  BitMask=65535  BitMaskRealWorld=Stored Integer
  BMS4_InputVolCHG_O : Constant  Value=0  OutDataTypeStr=single
  BMS4_InputVolCHG_S : ArithShift
  BMS4_InputVolCHG_Sub : Subsystem
  BMS4_InputVolCHG_sat : Saturate  UpperLimit=6553.5  LowerLimit=0
  BMS4_InputVolCHGcv : DataTypeConversion
  BMS4_InputVolCHGinput6_Ad : Sum
  BMS4_InputVolCHGinput6_C : Constant  Value=256
  BMS4_InputVolCHGinput6_P : Product
  BMS4_InputVolKEYON_Ad : Sum
  BMS4_InputVolKEYON_Convert : DataTypeConversion  OutDataTypeStr=uint32
  BMS4_InputVolKEYON_F : Gain  Gain=0.1
  BMS4_InputVolKEYON_L : simulink/Logic and Bit Operations/Bitwise Operator  logicop=AND  UseBitMask=on  BitMask=65535  BitMaskRealWorld=Stored Integer
  BMS4_InputVolKEYON_O : Constant  Value=0  OutDataTypeStr=single
  BMS4_InputVolKEYON_S : ArithShift
  BMS4_InputVolKEYON_Sub : Subsystem
  BMS4_InputVolKEYON_sat : Saturate  UpperLimit=6553.5  LowerLimit=0
  BMS4_InputVolKEYONcv : DataTypeConversion
  BMS4_InputVolKEYONinput4_Ad : Sum
  BMS4_InputVolKEYONinput4_C : Constant  Value=256
  BMS4_InputVolKEYONinput4_P : Product
  BMS4_Sys_Status3_Ad : Sum
  BMS4_Sys_Status3_Convert : DataTypeConversion  OutDataTypeStr=uint32
  BMS4_Sys_Status3_F : Gain
  BMS4_Sys_Status3_L : simulink/Logic and Bit Operations/Bitwise Operator  logicop=AND  UseBitMask=on  BitMask=255  BitMaskRealWorld=Stored Integer
  BMS4_Sys_Status3_O : Constant  Value=0  OutDataTypeStr=single
  BMS4_Sys_Status3_S : ArithShift
  BMS4_Sys_Status3_Sub : Subsystem
  BMS4_Sys_Status3_sat : Saturate  UpperLimit=255  LowerLimit=0
  BMS4_Sys_Status3cv : DataTypeConversion
  Demux : Demux  Outputs=8
  BMS4_Sys_Status3_Out : Outport
  BMS4_InputVolKEYON_Out : Outport  Port=2
  BMS4_InputVolCHG_Out : Outport  Port=3
  BMS4_InputVolACC_Out : Outport  Port=4
  wires:
  BMS4_Sys_Status3_F/1 -> BMS4_Sys_Status3_Ad/1
  BMS4_Sys_Status3_O/1 -> BMS4_Sys_Status3_Ad/2
  BMS4_Sys_Status3_Ad/1 -> BMS4_Sys_Status3_sat/1
  BMS4_Sys_Status3_sat/1 -> BMS4_Sys_Status3_Out/1
  Demux/1 -> BMS4_Sys_Status3_Sub/1(In1)
  BMS4_Sys_Status3_Sub/1(Out1) -> BMS4_Sys_Status3_Convert/1
  BMS4_Sys_Status3_Convert/1 -> BMS4_Sys_Status3_L/1
  BMS4_Sys_Status3_L/1 -> BMS4_Sys_Status3_S/1
  BMS4_Sys_Status3_S/1 -> BMS4_Sys_Status3cv/1
  BMS4_Sys_Status3cv/1 -> BMS4_Sys_Status3_F/1
  BMS4_InputVolKEYON_F/1 -> BMS4_InputVolKEYON_Ad/1
  BMS4_InputVolKEYON_O/1 -> BMS4_InputVolKEYON_Ad/2
  BMS4_InputVolKEYON_Ad/1 -> BMS4_InputVolKEYON_sat/1
  BMS4_InputVolKEYON_sat/1 -> BMS4_InputVolKEYON_Out/1
  Demux/4 -> BMS4_InputVolKEYONinput4_P/1
  BMS4_InputVolKEYONinput4_C/1 -> BMS4_InputVolKEYONinput4_P/2
  BMS4_InputVolKEYONinput4_P/1 -> BMS4_InputVolKEYONinput4_Ad/1
  Demux/5 -> BMS4_InputVolKEYONinput4_Ad/2
  BMS4_InputVolKEYONinput4_Ad/1 -> BMS4_InputVolKEYON_Sub/1(In1)
  BMS4_InputVolKEYON_Sub/1(Out1) -> BMS4_InputVolKEYON_Convert/1
  BMS4_InputVolKEYON_Convert/1 -> BMS4_InputVolKEYON_L/1
  BMS4_InputVolKEYON_L/1 -> BMS4_InputVolKEYON_S/1
  BMS4_InputVolKEYON_S/1 -> BMS4_InputVolKEYONcv/1
  BMS4_InputVolKEYONcv/1 -> BMS4_InputVolKEYON_F/1
  BMS4_InputVolCHG_F/1 -> BMS4_InputVolCHG_Ad/1
  BMS4_InputVolCHG_O/1 -> BMS4_InputVolCHG_Ad/2
  BMS4_InputVolCHG_Ad/1 -> BMS4_InputVolCHG_sat/1
  BMS4_InputVolCHG_sat/1 -> BMS4_InputVolCHG_Out/1
  Demux/6 -> BMS4_InputVolCHGinput6_P/1
  BMS4_InputVolCHGinput6_C/1 -> BMS4_InputVolCHGinput6_P/2
  BMS4_InputVolCHGinput6_P/1 -> BMS4_InputVolCHGinput6_Ad/1
  Demux/7 -> BMS4_InputVolCHGinput6_Ad/2
  BMS4_InputVolCHGinput6_Ad/1 -> BMS4_InputVolCHG_Sub/1(In1)
  BMS4_InputVolCHG_Sub/1(Out1) -> BMS4_InputVolCHG_Convert/1
  BMS4_InputVolCHG_Convert/1 -> BMS4_InputVolCHG_L/1
  BMS4_InputVolCHG_L/1 -> BMS4_InputVolCHG_S/1
  BMS4_InputVolCHG_S/1 -> BMS4_InputVolCHGcv/1
  BMS4_InputVolCHGcv/1 -> BMS4_InputVolCHG_F/1
  BMS4_InputVolACC_F/1 -> BMS4_InputVolACC_Ad/1
  BMS4_InputVolACC_O/1 -> BMS4_InputVolACC_Ad/2
  BMS4_InputVolACC_Ad/1 -> BMS4_InputVolACC_sat/1
  BMS4_InputVolACC_sat/1 -> BMS4_InputVolACC_Out/1
  Demux/2 -> BMS4_InputVolACCinput2_P/1
  BMS4_InputVolACCinput2_C/1 -> BMS4_InputVolACCinput2_P/2
  BMS4_InputVolACCinput2_P/1 -> BMS4_InputVolACCinput2_Ad/1
  Demux/3 -> BMS4_InputVolACCinput2_Ad/2
  BMS4_InputVolACCinput2_Ad/1 -> BMS4_InputVolACC_Sub/1(In1)
  BMS4_InputVolACC_Sub/1(Out1) -> BMS4_InputVolACC_Convert/1
  BMS4_InputVolACC_Convert/1 -> BMS4_InputVolACC_L/1
  BMS4_InputVolACC_L/1 -> BMS4_InputVolACC_S/1
  BMS4_InputVolACC_S/1 -> BMS4_InputVolACCcv/1
  BMS4_InputVolACCcv/1 -> BMS4_InputVolACC_F/1
  input/1 -> Demux/1

== matlab function six_plus_six_AcmsteeringV09_main_1lf/Data_input/5/Enabled Subsystem/MATLAB Function ==
  data: data1 input; y output; data2 input; data3 input; data4 input
function y = fcn(data1,data2,data3,data4)
%#codegen
y1=data4*256^3+data3*256^2+data2*256+data1;
y=typecast(uint32(y1),'single');
end
% y = u;

== matlab function six_plus_six_AcmsteeringV09_main_1lf/Data_input/7/Enabled Subsystem/MATLAB Function ==
  data: data1 input; y output; data2 input; data3 input; data4 input
function y = fcn(data1,data2,data3,data4)
%#codegen
y1=data4*256^3+data3*256^2+data2*256+data1;
y=typecast(uint32(y1),'single');
end
% y = u;

== matlab function six_plus_six_AcmsteeringV09_main_1lf/Data_input/9/Enabled Subsystem/MATLAB Function1 ==
  data: data1 input; y output; data2 input; data3 input; data4 input
function y = fcn(data1,data2,data3,data4)
%#codegen
y1=data4*256^3+data3*256^2+data2*256+data1;
% y=typecast(uint32(y1),'single');
y=single(y1*10^-7);
end
% y = u;

== matlab function six_plus_six_AcmsteeringV09_main_1lf/InputSignalProcess/MATLAB Function ==
  data: LeftJoystick_UpDown input; acc_dem output single; steer_dem output single; brake_dem output single; LeftJoystick_LeftRight input; RirhtJoystick_UpDown input
function [acc_dem,steer_dem,brake_dem] = fcn(LeftJoystick_UpDown,LeftJoystick_LeftRight,RirhtJoystick_UpDown)
%#codegen
if LeftJoystick_UpDown<=1512
    acc_dem=single((LeftJoystick_UpDown-1512)/(1094-1512)*100);
else
    acc_dem=single((LeftJoystick_UpDown-1512)/(1934-1512)*100*-1);
end

if  LeftJoystick_LeftRight <500 || LeftJoystick_LeftRight >2500
    steer_dem = single(0);
elseif LeftJoystick_LeftRight<=1503
    steer_dem=single((LeftJoystick_LeftRight-1503)/(1084-1503)*100);
else
    steer_dem=single((LeftJoystick_LeftRight-1503)/(1923-1503)*100*-1);
end

brake_dem=single((RirhtJoystick_UpDown-1094)/(1934-1094)*100);

end

== system six_plus_six_AcmsteeringV09_main_1lf/Data_input/BMS4_2/BMS4 ==
  input : Inport
  Enable : EnablePort
  BMS4_InputVolACC_Ad : Sum
  BMS4_InputVolACC_Convert : DataTypeConversion  OutDataTypeStr=uint32
  BMS4_InputVolACC_F : Gain  Gain=0.1
  BMS4_InputVolACC_L : simulink/Logic and Bit Operations/Bitwise Operator  logicop=AND  UseBitMask=on  BitMask=65535  BitMaskRealWorld=Stored Integer
  BMS4_InputVolACC_O : Constant  Value=0  OutDataTypeStr=single
  BMS4_InputVolACC_S : ArithShift
  BMS4_InputVolACC_Sub : Subsystem
  BMS4_InputVolACC_sat : Saturate  UpperLimit=6553.5  LowerLimit=0
  BMS4_InputVolACCcv : DataTypeConversion
  BMS4_InputVolACCinput2_Ad : Sum
  BMS4_InputVolACCinput2_C : Constant  Value=256
  BMS4_InputVolACCinput2_P : Product
  BMS4_InputVolCHG_Ad : Sum
  BMS4_InputVolCHG_Convert : DataTypeConversion  OutDataTypeStr=uint32
  BMS4_InputVolCHG_F : Gain  Gain=0.1
  BMS4_InputVolCHG_L : simulink/Logic and Bit Operations/Bitwise Operator  logicop=AND  UseBitMask=on  BitMask=65535  BitMaskRealWorld=Stored Integer
  BMS4_InputVolCHG_O : Constant  Value=0  OutDataTypeStr=single
  BMS4_InputVolCHG_S : ArithShift
  BMS4_InputVolCHG_Sub : Subsystem
  BMS4_InputVolCHG_sat : Saturate  UpperLimit=6553.5  LowerLimit=0
  BMS4_InputVolCHGcv : DataTypeConversion
  BMS4_InputVolCHGinput6_Ad : Sum
  BMS4_InputVolCHGinput6_C : Constant  Value=256
  BMS4_InputVolCHGinput6_P : Product
  BMS4_InputVolKEYON_Ad : Sum
  BMS4_InputVolKEYON_Convert : DataTypeConversion  OutDataTypeStr=uint32
  BMS4_InputVolKEYON_F : Gain  Gain=0.1
  BMS4_InputVolKEYON_L : simulink/Logic and Bit Operations/Bitwise Operator  logicop=AND  UseBitMask=on  BitMask=65535  BitMaskRealWorld=Stored Integer
  BMS4_InputVolKEYON_O : Constant  Value=0  OutDataTypeStr=single
  BMS4_InputVolKEYON_S : ArithShift
  BMS4_InputVolKEYON_Sub : Subsystem
  BMS4_InputVolKEYON_sat : Saturate  UpperLimit=6553.5  LowerLimit=0
  BMS4_InputVolKEYONcv : DataTypeConversion
  BMS4_InputVolKEYONinput4_Ad : Sum
  BMS4_InputVolKEYONinput4_C : Constant  Value=256
  BMS4_InputVolKEYONinput4_P : Product
  BMS4_Sys_Status3_Ad : Sum
  BMS4_Sys_Status3_Convert : DataTypeConversion  OutDataTypeStr=uint32
  BMS4_Sys_Status3_F : Gain
  BMS4_Sys_Status3_L : simulink/Logic and Bit Operations/Bitwise Operator  logicop=AND  UseBitMask=on  BitMask=255  BitMaskRealWorld=Stored Integer
  BMS4_Sys_Status3_O : Constant  Value=0  OutDataTypeStr=single
  BMS4_Sys_Status3_S : ArithShift
  BMS4_Sys_Status3_Sub : Subsystem
  BMS4_Sys_Status3_sat : Saturate  UpperLimit=255  LowerLimit=0
  BMS4_Sys_Status3cv : DataTypeConversion
  Demux : Demux  Outputs=8
  BMS4_Sys_Status3_Out : Outport
  BMS4_InputVolKEYON_Out : Outport  Port=2
  BMS4_InputVolCHG_Out : Outport  Port=3
  BMS4_InputVolACC_Out : Outport  Port=4
  wires:
  BMS4_Sys_Status3_F/1 -> BMS4_Sys_Status3_Ad/1
  BMS4_Sys_Status3_O/1 -> BMS4_Sys_Status3_Ad/2
  BMS4_Sys_Status3_Ad/1 -> BMS4_Sys_Status3_sat/1
  BMS4_Sys_Status3_sat/1 -> BMS4_Sys_Status3_Out/1
  Demux/1 -> BMS4_Sys_Status3_Sub/1(In1)
  BMS4_Sys_Status3_Sub/1(Out1) -> BMS4_Sys_Status3_Convert/1
  BMS4_Sys_Status3_Convert/1 -> BMS4_Sys_Status3_L/1
  BMS4_Sys_Status3_L/1 -> BMS4_Sys_Status3_S/1
  BMS4_Sys_Status3_S/1 -> BMS4_Sys_Status3cv/1
  BMS4_Sys_Status3cv/1 -> BMS4_Sys_Status3_F/1
  BMS4_InputVolKEYON_F/1 -> BMS4_InputVolKEYON_Ad/1
  BMS4_InputVolKEYON_O/1 -> BMS4_InputVolKEYON_Ad/2
  BMS4_InputVolKEYON_Ad/1 -> BMS4_InputVolKEYON_sat/1
  BMS4_InputVolKEYON_sat/1 -> BMS4_InputVolKEYON_Out/1
  Demux/4 -> BMS4_InputVolKEYONinput4_P/1
  BMS4_InputVolKEYONinput4_C/1 -> BMS4_InputVolKEYONinput4_P/2
  BMS4_InputVolKEYONinput4_P/1 -> BMS4_InputVolKEYONinput4_Ad/1
  Demux/5 -> BMS4_InputVolKEYONinput4_Ad/2
  BMS4_InputVolKEYONinput4_Ad/1 -> BMS4_InputVolKEYON_Sub/1(In1)
  BMS4_InputVolKEYON_Sub/1(Out1) -> BMS4_InputVolKEYON_Convert/1
  BMS4_InputVolKEYON_Convert/1 -> BMS4_InputVolKEYON_L/1
  BMS4_InputVolKEYON_L/1 -> BMS4_InputVolKEYON_S/1
  BMS4_InputVolKEYON_S/1 -> BMS4_InputVolKEYONcv/1
  BMS4_InputVolKEYONcv/1 -> BMS4_InputVolKEYON_F/1
  BMS4_InputVolCHG_F/1 -> BMS4_InputVolCHG_Ad/1
  BMS4_InputVolCHG_O/1 -> BMS4_InputVolCHG_Ad/2
  BMS4_InputVolCHG_Ad/1 -> BMS4_InputVolCHG_sat/1
  BMS4_InputVolCHG_sat/1 -> BMS4_InputVolCHG_Out/1
  Demux/6 -> BMS4_InputVolCHGinput6_P/1
  BMS4_InputVolCHGinput6_C/1 -> BMS4_InputVolCHGinput6_P/2
  BMS4_InputVolCHGinput6_P/1 -> BMS4_InputVolCHGinput6_Ad/1
  Demux/7 -> BMS4_InputVolCHGinput6_Ad/2
  BMS4_InputVolCHGinput6_Ad/1 -> BMS4_InputVolCHG_Sub/1(In1)
  BMS4_InputVolCHG_Sub/1(Out1) -> BMS4_InputVolCHG_Convert/1
  BMS4_InputVolCHG_Convert/1 -> BMS4_InputVolCHG_L/1
  BMS4_InputVolCHG_L/1 -> BMS4_InputVolCHG_S/1
  BMS4_InputVolCHG_S/1 -> BMS4_InputVolCHGcv/1
  BMS4_InputVolCHGcv/1 -> BMS4_InputVolCHG_F/1
  BMS4_InputVolACC_F/1 -> BMS4_InputVolACC_Ad/1
  BMS4_InputVolACC_O/1 -> BMS4_InputVolACC_Ad/2
  BMS4_InputVolACC_Ad/1 -> BMS4_InputVolACC_sat/1
  BMS4_InputVolACC_sat/1 -> BMS4_InputVolACC_Out/1
  Demux/2 -> BMS4_InputVolACCinput2_P/1
  BMS4_InputVolACCinput2_C/1 -> BMS4_InputVolACCinput2_P/2
  BMS4_InputVolACCinput2_P/1 -> BMS4_InputVolACCinput2_Ad/1
  Demux/3 -> BMS4_InputVolACCinput2_Ad/2
  BMS4_InputVolACCinput2_Ad/1 -> BMS4_InputVolACC_Sub/1(In1)
  BMS4_InputVolACC_Sub/1(Out1) -> BMS4_InputVolACC_Convert/1
  BMS4_InputVolACC_Convert/1 -> BMS4_InputVolACC_L/1
  BMS4_InputVolACC_L/1 -> BMS4_InputVolACC_S/1
  BMS4_InputVolACC_S/1 -> BMS4_InputVolACCcv/1
  BMS4_InputVolACCcv/1 -> BMS4_InputVolACC_F/1
  input/1 -> Demux/1
